simulink model "FourBitAdder_Block"  (R2024a)
settings: Solver=ode45  StartTime=0.0  StopTime=inf  RelTol=1e-3  EnableMultiTasking=on
settings Model: Creator=nunkesser  LastModifiedBy=nunkesser
settings SolverCC: AlgebraicLoopSolver=TrustRegion
settings DataIOCC: LimitDataPoints=on  SaveFormat=Array  ReturnWorkspaceOutputs=off
settings OptimizationCC: LifeSpan=inf
settings DebuggingCC: SolverPrmCheckMsg=warning  UnconnectedInputMsg=warning  UnconnectedOutputMsg=warning  UnconnectedLineMsg=warning  SFUnexpectedBacktrackingDiag=warning  SFNoUnconditionalDefaultTransitionDiag=warning  SFExecutionAtInitializationDiag=none  ArithmeticOperatorsInVariantConditions=warning
settings HardwareCC: ProdBitPerPointer=32  ProdBitPerSizeT=32  ProdBitPerPtrDiffT=32  ProdLargestAtomicFloat=None  ProdIntDivRoundTo=Undefined  ProdEndianess=Unspecified  ProdWordSize=32  ProdHWDeviceType=32-bit Generic
settings ModelReferenceCC: PropagateSignalLabelsOutOfModel=off
settings SFSimCC: SimUseLocalCustomCode=off  CustomCodeUndefinedFunction=UseInterfaceOnly
settings RTWCC: RTWUseLocalCustomCode=off  GPUComputeCapability=3.5
settings CodeAppCC: StateflowObjectComments=on
settings GRTTargetCC: TargetLangStandard=C89/C90 (ANSI)
settings ConfigComp: CovMetricSettings=dw  CovSaveCumulativeToWorkspaceVar=on  CovSaveSingleToWorkspaceVar=on  CovExternalEMLEnable=off  CovSFcnEnable=off

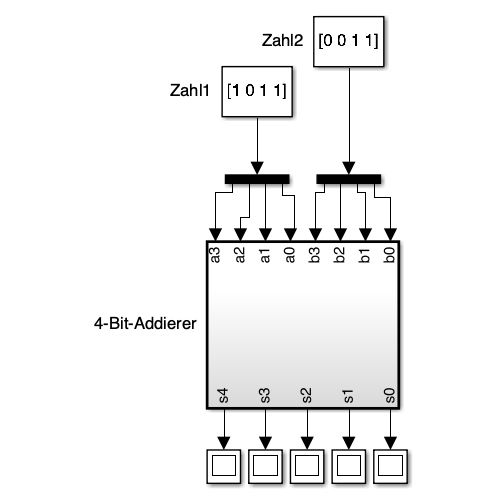
[thumbnail: Simulink's stored preview of the top-level diagram]
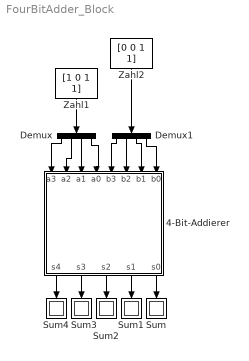
== system FourBitAdder_Block ==
  4-Bit-Addierer : Subsystem  TreatAsAtomicUnit=on
  Demux : Demux
  Demux1 : Demux
  Sum{,1..4} (5 alike) : Display
  Zahl1 : Constant  Value=[1 0 1 1]
  Zahl2 : Constant  Value=[0 0 1 1]
  wires:
  Zahl1/1 -> Demux/1
  Demux/4 -> 4-Bit-Addierer/4(a0)
  Zahl2/1 -> Demux1/1
  4-Bit-Addierer/5(s0) -> Sum/1
  Demux1/4 -> 4-Bit-Addierer/8(b0)
  4-Bit-Addierer/4(s1) -> Sum1/1
  Demux1/3 -> 4-Bit-Addierer/7(b1)
  Demux/3 -> 4-Bit-Addierer/3(a1)
  Demux1/2 -> 4-Bit-Addierer/6(b2)
  Demux/2 -> 4-Bit-Addierer/2(a2)
  4-Bit-Addierer/3(s2) -> Sum2/1
  Demux/1 -> 4-Bit-Addierer/1(a3)
  Demux1/1 -> 4-Bit-Addierer/5(b3)
  4-Bit-Addierer/2(s3) -> Sum3/1
  4-Bit-Addierer/1(s4) -> Sum4/1

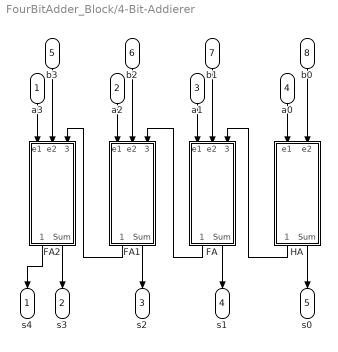
== system FourBitAdder_Block/4-Bit-Addierer ==
  a3 : Inport
  a2 : Inport  Port=2
  a1 : Inport  Port=3
  a0 : Inport  Port=4
  b3 : Inport  Port=5
  b2 : Inport  Port=6
  b1 : Inport  Port=7
  b0 : Inport  Port=8
  FA : Subsystem  TreatAsAtomicUnit=on
  FA1 : Subsystem  TreatAsAtomicUnit=on
  FA2 : Subsystem  TreatAsAtomicUnit=on
  HA : Subsystem  TreatAsAtomicUnit=on
  s4 : Outport
  s3 : Outport  Port=2
  s2 : Outport  Port=3
  s1 : Outport  Port=4
  s0 : Outport  Port=5
  wires:
  a0/1 -> HA/1(e1)
  HA/2(Sum) -> s0/1
  HA/1(Carry) -> FA/3(CarryIn)
  b0/1 -> HA/2(e2)
  FA/2(Sum) -> s1/1
  b1/1 -> FA/2(e2)
  a1/1 -> FA/1(e1)
  FA/1(CarryOut) -> FA1/3(CarryIn)
  b2/1 -> FA1/2(e2)
  a2/1 -> FA1/1(e1)
  FA1/2(Sum) -> s2/1
  FA1/1(CarryOut) -> FA2/3(CarryIn)
  a3/1 -> FA2/1(e1)
  b3/1 -> FA2/2(e2)
  FA2/2(Sum) -> s3/1
  FA2/1(CarryOut) -> s4/1

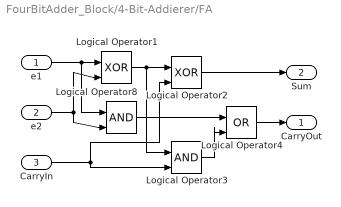
== system FourBitAdder_Block/4-Bit-Addierer/FA ==
  e1 : Inport
  e2 : Inport  Port=2
  CarryIn : Inport  Port=3
  Logical Operator1 : Logic  Operator=XOR  IconShape=distinctive  AllPortsSameDT=off  OutDataTypeStr=boolean
  Logical Operator2 : Logic  Operator=XOR  IconShape=distinctive  AllPortsSameDT=off  OutDataTypeStr=boolean
  Logical Operator3 : Logic  IconShape=distinctive  AllPortsSameDT=off  OutDataTypeStr=boolean
  Logical Operator4 : Logic  Operator=OR  IconShape=distinctive  AllPortsSameDT=off  OutDataTypeStr=boolean
  Logical Operator8 : Logic  IconShape=distinctive  AllPortsSameDT=off  OutDataTypeStr=boolean
  CarryOut : Outport
  Sum : Outport  Port=2
  wires:
  e2/1 -> Logical Operator8/2, Logical Operator1/2
  Logical Operator1/1 -> Logical Operator2/1, Logical Operator3/1
  CarryIn/1 -> Logical Operator2/2, Logical Operator3/2
  Logical Operator2/1 -> Sum/1
  Logical Operator8/1 -> Logical Operator4/1
  Logical Operator3/1 -> Logical Operator4/2
  Logical Operator4/1 -> CarryOut/1
  e1/1 -> Logical Operator8/1, Logical Operator1/1

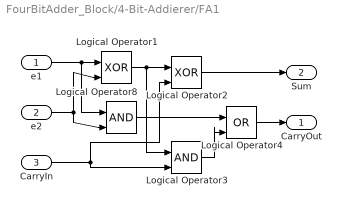
== system FourBitAdder_Block/4-Bit-Addierer/FA1 ==
  e1 : Inport
  e2 : Inport  Port=2
  CarryIn : Inport  Port=3
  Logical Operator1 : Logic  Operator=XOR  IconShape=distinctive  AllPortsSameDT=off  OutDataTypeStr=boolean
  Logical Operator2 : Logic  Operator=XOR  IconShape=distinctive  AllPortsSameDT=off  OutDataTypeStr=boolean
  Logical Operator3 : Logic  IconShape=distinctive  AllPortsSameDT=off  OutDataTypeStr=boolean
  Logical Operator4 : Logic  Operator=OR  IconShape=distinctive  AllPortsSameDT=off  OutDataTypeStr=boolean
  Logical Operator8 : Logic  IconShape=distinctive  AllPortsSameDT=off  OutDataTypeStr=boolean
  CarryOut : Outport
  Sum : Outport  Port=2
  wires:
  e2/1 -> Logical Operator8/2, Logical Operator1/2
  Logical Operator1/1 -> Logical Operator2/1, Logical Operator3/1
  CarryIn/1 -> Logical Operator2/2, Logical Operator3/2
  Logical Operator2/1 -> Sum/1
  Logical Operator8/1 -> Logical Operator4/1
  Logical Operator3/1 -> Logical Operator4/2
  Logical Operator4/1 -> CarryOut/1
  e1/1 -> Logical Operator8/1, Logical Operator1/1

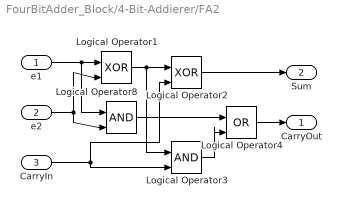
== system FourBitAdder_Block/4-Bit-Addierer/FA2 ==
  e1 : Inport
  e2 : Inport  Port=2
  CarryIn : Inport  Port=3
  Logical Operator1 : Logic  Operator=XOR  IconShape=distinctive  AllPortsSameDT=off  OutDataTypeStr=boolean
  Logical Operator2 : Logic  Operator=XOR  IconShape=distinctive  AllPortsSameDT=off  OutDataTypeStr=boolean
  Logical Operator3 : Logic  IconShape=distinctive  AllPortsSameDT=off  OutDataTypeStr=boolean
  Logical Operator4 : Logic  Operator=OR  IconShape=distinctive  AllPortsSameDT=off  OutDataTypeStr=boolean
  Logical Operator8 : Logic  IconShape=distinctive  AllPortsSameDT=off  OutDataTypeStr=boolean
  CarryOut : Outport
  Sum : Outport  Port=2
  wires:
  e2/1 -> Logical Operator8/2, Logical Operator1/2
  Logical Operator1/1 -> Logical Operator2/1, Logical Operator3/1
  CarryIn/1 -> Logical Operator2/2, Logical Operator3/2
  Logical Operator2/1 -> Sum/1
  Logical Operator8/1 -> Logical Operator4/1
  Logical Operator3/1 -> Logical Operator4/2
  Logical Operator4/1 -> CarryOut/1
  e1/1 -> Logical Operator8/1, Logical Operator1/1

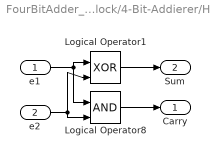
== system FourBitAdder_Block/4-Bit-Addierer/HA ==
  e1 : Inport
  e2 : Inport  Port=2
  Logical Operator1 : Logic  Operator=XOR  IconShape=distinctive  AllPortsSameDT=off  OutDataTypeStr=boolean
  Logical Operator8 : Logic  IconShape=distinctive  AllPortsSameDT=off  OutDataTypeStr=boolean
  Carry : Outport
  Sum : Outport  Port=2
  wires:
  e1/1 -> Logical Operator1/1, Logical Operator8/1
  e2/1 -> Logical Operator1/2, Logical Operator8/2
  Logical Operator1/1 -> Sum/1
  Logical Operator8/1 -> Carry/1
